simulink model "untitled"  (R2017b)
settings: Solver=VariableStepAuto  StartTime=0.0  StopTime=200.0  RelTol=1e-3
settings Model: Creator=piopi  LastModifiedBy=piopi

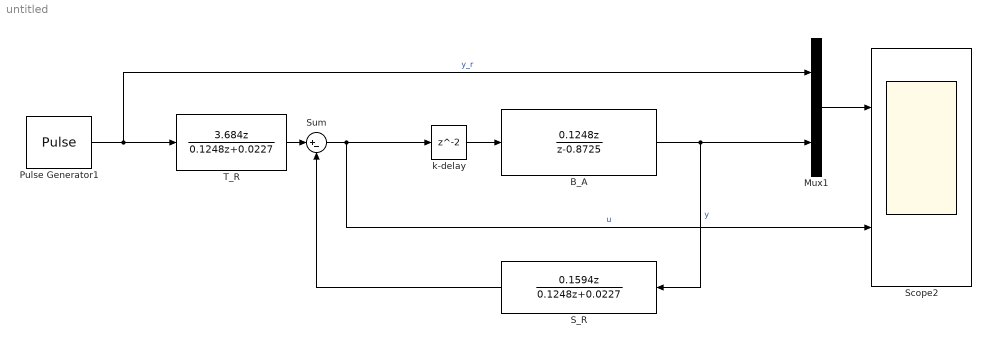
== system untitled ==
  B_A : DiscreteTransferFcn  Numerator=[0.1248 0]  Denominator=[1 -0.8725]  SampleTime=2
  Mux1 : Mux  Inputs=2
  Pulse Generator1 : DiscretePulseGenerator  PulseType=Time based  Period=240  PulseWidth=50
  S_R : DiscreteTransferFcn  Numerator=[0.1594 0]  Denominator=[0.1248, 0.0227]  SampleTime=2
  Scope2 : Scope  NumInputPorts=2
  Sum : Sum  Inputs=|+-
  T_R : DiscreteTransferFcn  Numerator=[3.684 0]  Denominator=[0.1248, 0.0227]  SampleTime=2
  k-delay : Delay  SampleTime=2
  wires:
  Sum/1 -> k-delay/1, Scope2/2  "u"
  Pulse Generator1/1 -> Mux1/1, T_R/1  "y_r"
  B_A/1 -> Mux1/2, S_R/1  "y"
  Mux1/1 -> Scope2/1
  T_R/1 -> Sum/1
  S_R/1 -> Sum/2
  k-delay/1 -> B_A/1
